simulink model "Sim2_test_cor_PI"  (R2018b)
settings: Solver=ode1  StartTime=0.0  StopTime=2  FixedStep=Time_Step  MaxStep=1e-4  RelTol=1e-3
undefined symbols (not defined in the file): abc2dq0_norm, Control_Lib, dq02abc_norm, Lg, PLL, Rg, Theta0, Time_Step, Ug, Un, V0, VSC01_id0
libraries: powerlib x35, simulink x17
(part 3 of 3)

== system Sim2_test_cor_PI/VSC02/Control loops/abc2dq0_norm1 ==
  abc : Inport
  CosSinTheta : Inport  Port=2
  Add : Sum
  Add1 : Sum  Inputs=-+
  Compare To Constant : simulink/Logic and Bit Operations/Compare To Constant  relop===  const=1  OutDataTypeStr=boolean
  Constant : Constant  Value=referenceAxisMode  OutDataTypeStr=uint16
  Demux : Demux  Outputs=2
  Demux1 : Demux  Outputs=3
  Gain : Gain  Gain=Concordia33  Multiplication=Matrix(K*u)
  Gain1 : Gain  Gain=baseUpdateGain
  Mux : Mux  Inputs=2
  Product{,1..3} (4 alike) : Product
  RotationInv90Deg : Subsystem  VariantControl=ROTATIONINV90DEG
  Switch : Switch  Criteria=u2 ~= 0
  AlphaBeta : Outport  VectorParamsAs1DForOutWhenUnconnected=off
  dq : Outport  Port=2  VectorParamsAs1DForOutWhenUnconnected=off
  ZeroSequence : Outport  Port=3  VectorParamsAs1DForOutWhenUnconnected=off
  wires:
  Gain1/1 -> Gain/1
  Compare To Constant/1 -> Switch/2
  Constant/1 -> Compare To Constant/1
  RotationInv90Deg/1(CosSinThetaOut) -> Switch/3
  CosSinTheta/1 -> RotationInv90Deg/1(CosSinThetaIn), Switch/1
  Switch/1 -> Demux/1
  Demux/1 -> Product/2, Product3/2
  Product3/1 -> Add1/2
  Product1/1 -> Add/2
  Demux/2 -> Product1/2, Product2/2
  Add1/1 -> Mux/2
  Gain/1 -> Demux1/1, AlphaBeta/1
  Demux1/2 -> Product3/1, Product1/1  "beta"
  Mux/1 -> dq/1
  Demux1/3 -> ZeroSequence/1  "zero"
  Add/1 -> Mux/1
  Demux1/1 -> Product2/1, Product/1  "alpha"
  Product/1 -> Add/1
  Product2/1 -> Add1/1
  abc/1 -> Gain1/1

== system Sim2_test_cor_PI/VSC02/Control loops/dq02abc_norm ==
  dq : Inport
  ZeroSequence : Inport  Port=2
  CosSinTheta : Inport  Port=3
  Add : Sum  Inputs=+-
  Add1 : Sum
  Compare To Constant : simulink/Logic and Bit Operations/Compare To Constant  relop===  const=1  OutDataTypeStr=boolean
  Constant : Constant  Value=referenceAxisMode  OutDataTypeStr=uint16
  Demux : Demux  Outputs=2
  Demux2 : Demux  Outputs=2
  Gain : Gain  Gain=Concordia33_inv  Multiplication=Matrix(K*u)
  Gain1 : Gain  Gain=baseUpdateGain
  Mux : Mux  Inputs=3
  Mux1 : Mux  Inputs=2
  Product{,1..3} (4 alike) : Product
  RotationInv90Deg : Subsystem  VariantControl=ROTATIONINV90DEG
  Switch : Switch  Criteria=u2 ~= 0
  AlphaBeta : Outport  VectorParamsAs1DForOutWhenUnconnected=off
  abc : Outport  Port=2  VectorParamsAs1DForOutWhenUnconnected=off
  wires:
  Gain1/1 -> abc/1
  Constant/1 -> Compare To Constant/1
  RotationInv90Deg/1(CosSinThetaOut) -> Switch/3
  Demux/1 -> Product3/2, Product/2
  Mux/1 -> Gain/1
  Switch/1 -> Demux/1
  Demux/2 -> Product2/2, Product1/2
  Mux1/1 -> AlphaBeta/1
  Product/1 -> Add/1
  Demux2/2 -> Product1/1, Product3/1  "q"
  Add1/1 -> Mux/2, Mux1/2  "beta"
  Product1/1 -> Add/2
  Compare To Constant/1 -> Switch/2
  Product2/1 -> Add1/1
  Product3/1 -> Add1/2
  CosSinTheta/1 -> Switch/1, RotationInv90Deg/1(CosSinThetaIn)
  dq/1 -> Demux2/1
  ZeroSequence/1 -> Mux/3
  Demux2/1 -> Product/1, Product2/1  "d"
  Add/1 -> Mux/1, Mux1/1  "alpha"
  Gain/1 -> Gain1/1

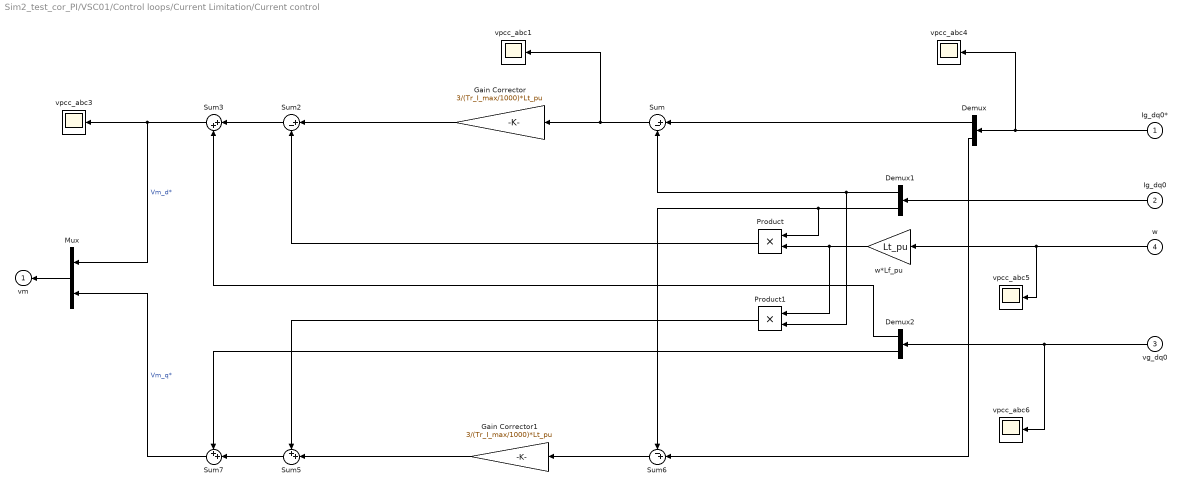
== system Sim2_test_cor_PI/VSC01/Control loops/Current Limitation/Current control ==
  Ig_dq0* : Inport
  Ig_dq0 : Inport  Port=2
  vg_dq0 : Inport  Port=3
  w : Inport  Port=4
  Demux : Demux  Outputs=2
  Demux1 : Demux  Outputs=2
  Demux2 : Demux  Outputs=2
  Gain Corrector : Gain  Gain=3/(Tr_I_max/1000)*Lt_pu
  Gain Corrector1 : Gain  Gain=3/(Tr_I_max/1000)*Lt_pu
  Mux : Mux  Inputs=2
  Product : Product  RndMeth=Zero
  Product1 : Product  RndMeth=Zero
  Sum : Sum  Inputs=|+-
  Sum2 : Sum  Inputs=|+-
  Sum3 : Sum  Inputs=|++
  Sum5 : Sum  Inputs=++|
  Sum6 : Sum  Inputs=-+|
  Sum7 : Sum  Inputs=++|
  vpcc_abc{1,3..6} (5 alike) : Scope
  w*Lf_pu : Gain  Gain=Lt_pu
  vm : Outport  InitialOutput=0  VectorParamsAs1DForOutWhenUnconnected=off
  wires:
  Demux2/2 -> Sum7/1
  Demux2/1 -> Sum3/2
  w/1 -> vpcc_abc5/1, w*Lf_pu/1
  Sum/1 -> vpcc_abc1/1, Gain Corrector/1
  Sum7/1 -> Mux/2  "Vm_q*"
  Sum3/1 -> Mux/1, vpcc_abc3/1  "Vm_d*"
  Sum5/1 -> Sum7/2
  Product1/1 -> Sum5/1
  Gain Corrector1/1 -> Sum5/2
  Demux/2 -> Sum6/2
  Sum2/1 -> Sum3/1
  Product/1 -> Sum2/2
  Demux1/2 -> Sum6/1, Product/1
  w*Lf_pu/1 -> Product/2, Product1/1
  Gain Corrector/1 -> Sum2/1
  Demux1/1 -> Sum/2, Product1/2
  Demux/1 -> Sum/1
  Ig_dq0/1 -> Demux1/1
  vg_dq0/1 -> Demux2/1, vpcc_abc6/1
  Sum6/1 -> Gain Corrector1/1
  Ig_dq0*/1 -> vpcc_abc4/1, Demux/1
  Mux/1 -> vm/1

== system Sim2_test_cor_PI/VSC01/Control loops/Current Limitation/Inverse Current control ==
  Vm_dq* : Inport
  Ig_dq : Inport  Port=2
  vg_dq : Inport  Port=3
  w : Inport  Port=4
  Demux : Demux  Outputs=2
  Demux1 : Demux  Outputs=2
  Demux2 : Demux  Outputs=2
  Gain Corrector2 : Gain  Gain=1/(3/(Tr_I_max/1000)*Lt_pu)
  Gain Corrector3 : Gain  Gain=1/(3/(Tr_I_max/1000)*Lt_pu)
  Mux : Mux  Inputs=2
  Product : Product  RndMeth=Zero
  Product1 : Product  RndMeth=Zero
  Sum : Sum  Inputs=|+-
  Sum2 : Sum  Inputs=|++
  Sum3 : Sum  Inputs=|++
  Sum5 : Sum  Inputs=-+|
  Sum6 : Sum  Inputs=-+|
  Sum7 : Sum  Inputs=++|
  w*Lf_pu : Gain  Gain=Lt_pu
  Is_dq* : Outport  InitialOutput=0  VectorParamsAs1DForOutWhenUnconnected=off
  wires:
  vg_dq/1 -> Demux2/1
  Ig_dq/1 -> Demux1/1
  Vm_dq*/1 -> Demux/1
  Demux/1 -> Sum/1
  Demux1/1 -> Sum3/2, Product1/2
  Sum/1 -> Sum2/1
  w*Lf_pu/1 -> Product1/1, Product/2
  Product/1 -> Sum2/2
  Sum2/1 -> Gain Corrector3/1
  Mux/1 -> Is_dq*/1
  Demux/2 -> Sum6/2
  Sum6/1 -> Sum5/2
  Sum5/1 -> Gain Corrector2/1
  Sum3/1 -> Mux/1  "is_d*"
  Sum7/1 -> Mux/2  "is_q*"
  w/1 -> w*Lf_pu/1
  Demux1/2 -> Sum7/1, Product/1
  Gain Corrector3/1 -> Sum3/1
  Demux2/1 -> Sum/2
  Demux2/2 -> Sum6/1
  Product1/1 -> Sum5/1
  Gain Corrector2/1 -> Sum7/2

== system Sim2_test_cor_PI/VSC01/Control loops/PLL/PI PLL controller ==
  vq : Inport
  0 - Vd1 : Gain  Gain=Kp_PLL  SaturateOnIntegerOverflow=on  OutDataTypeStr=Inherit: Same as input  ParamDataTypeStr=Inherit: Same as input
  0 - Vd2 : Gain  Gain=Ki_PLL  SaturateOnIntegerOverflow=on  OutDataTypeStr=Inherit: Same as input  ParamDataTypeStr=Inherit: Same as input
  Integrator : Integrator
  Integrator1 : Integrator  InitialCondition=Theta0*pi/180
  Sum : Sum  SaturateOnIntegerOverflow=on
  Sum1 : Sum  SaturateOnIntegerOverflow=on
  w_PLL_pu : Gain  Gain=wb  SaturateOnIntegerOverflow=on  OutDataTypeStr=Inherit: Same as input  ParamDataTypeStr=Inherit: Same as input
  w_set : Constant
  w : Outport  VectorParamsAs1DForOutWhenUnconnected=off
  Theta : Outport  Port=2  VectorParamsAs1DForOutWhenUnconnected=off
  wires:
  Integrator1/1 -> Theta/1
  0 - Vd2/1 -> Integrator/1
  w_set/1 -> Sum1/1
  w_PLL_pu/1 -> Integrator1/1
  Integrator/1 -> Sum/2
  Sum/1 -> Sum1/2
  0 - Vd1/1 -> Sum/1
  vq/1 -> 0 - Vd2/1, 0 - Vd1/1
  Sum1/1 -> w/1, w_PLL_pu/1

== system Sim2_test_cor_PI/VSC01/Control loops/PLL/abc2dq0_norm ==
  abc : Inport
  CosSinTheta : Inport  Port=2
  Add : Sum
  Add1 : Sum  Inputs=-+
  Compare To Constant : simulink/Logic and Bit Operations/Compare To Constant  relop===  const=1  OutDataTypeStr=boolean
  Constant : Constant  Value=referenceAxisMode  OutDataTypeStr=uint16
  Demux : Demux  Outputs=2
  Demux1 : Demux  Outputs=3
  Gain : Gain  Gain=Concordia33  Multiplication=Matrix(K*u)
  Gain1 : Gain  Gain=baseUpdateGain
  Mux : Mux  Inputs=2
  Product{,1..3} (4 alike) : Product
  RotationInv90Deg : Subsystem  VariantControl=ROTATIONINV90DEG
  Switch : Switch  Criteria=u2 ~= 0
  AlphaBeta : Outport  VectorParamsAs1DForOutWhenUnconnected=off
  dq : Outport  Port=2  VectorParamsAs1DForOutWhenUnconnected=off
  ZeroSequence : Outport  Port=3  VectorParamsAs1DForOutWhenUnconnected=off
  wires:
  Gain1/1 -> Gain/1
  Compare To Constant/1 -> Switch/2
  Constant/1 -> Compare To Constant/1
  RotationInv90Deg/1(CosSinThetaOut) -> Switch/3
  CosSinTheta/1 -> RotationInv90Deg/1(CosSinThetaIn), Switch/1
  Switch/1 -> Demux/1
  Demux/1 -> Product/2, Product3/2
  Product3/1 -> Add1/2
  Product1/1 -> Add/2
  Demux/2 -> Product1/2, Product2/2
  Add1/1 -> Mux/2
  Gain/1 -> Demux1/1, AlphaBeta/1
  Demux1/2 -> Product3/1, Product1/1  "beta"
  Mux/1 -> dq/1
  Demux1/3 -> ZeroSequence/1  "zero"
  Add/1 -> Mux/1
  Demux1/1 -> Product2/1, Product/1  "alpha"
  Product/1 -> Add/1
  Product2/1 -> Add1/1
  abc/1 -> Gain1/1

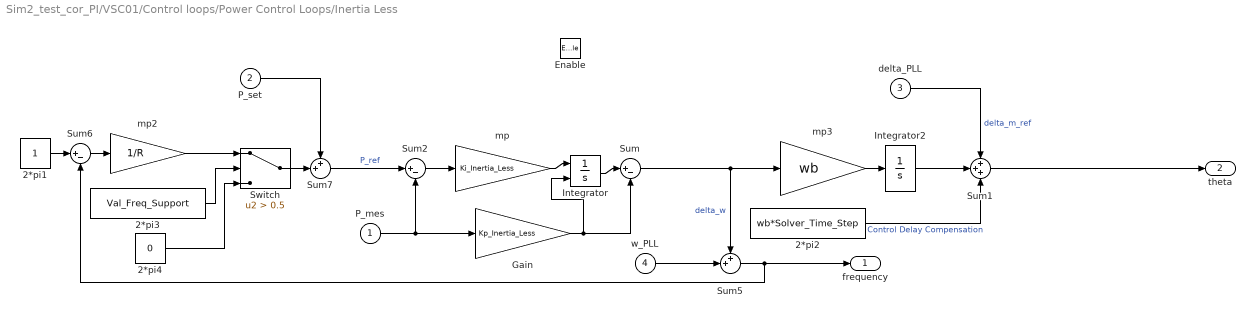
== system Sim2_test_cor_PI/VSC01/Control loops/Power Control Loops/Inertia Less ==
  P_mes : Inport
  P_set : Inport  Port=2
  delta_PLL : Inport  Port=3
  w_PLL : Inport  Port=4
  Enable : EnablePort
  2*pi1 : Constant
  2*pi2 : Constant  Value=wb*Solver_Time_Step
  2*pi3 : Constant  Value=Val_Freq_Support
  2*pi4 : Constant  Value=0
  Gain : Gain  Gain=Kp_Inertia_Less
  Integrator : Integrator  InitialConditionSource=external
  Integrator2 : Integrator  InitialCondition=(Theta_vsc0)*pi/180-Theta0*pi/180
  Sum : Sum  Inputs=|+-
  Sum1 : Sum  Inputs=+++
  Sum2 : Sum  Inputs=|+-
  Sum5 : Sum  Inputs=++|
  Sum6 : Sum  Inputs=|+-
  Sum7 : Sum  Inputs=++|
  Switch : Switch  Criteria=u2 > Threshold  Threshold=0.5
  mp : Gain  Gain=Ki_Inertia_Less
  mp2 : Gain  Gain=1/R
  mp3 : Gain  Gain=wb
  frequency : Outport  VectorParamsAs1DForOutWhenUnconnected=off
  theta : Outport  Port=2  VectorParamsAs1DForOutWhenUnconnected=off
  wires:
  Gain/1 -> Sum/2, Integrator/2
  Integrator/1 -> Sum/1
  2*pi4/1 -> Switch/3
  2*pi3/1 -> Switch/2
  mp2/1 -> Switch/1
  Integrator2/1 -> Sum1/2
  2*pi2/1 -> Sum1/3  "Control Delay Compensation"
  Sum5/1 -> Sum6/2, frequency/1
  w_PLL/1 -> Sum5/2
  delta_PLL/1 -> Sum1/1  "delta_m_ref"
  mp/1 -> Integrator/1
  mp3/1 -> Integrator2/1
  Sum/1 -> Sum5/1, mp3/1  "delta_w"
  Sum1/1 -> theta/1
  Switch/1 -> Sum7/2
  P_mes/1 -> Sum2/2, Gain/1
  Sum7/1 -> Sum2/1  "P_ref"
  P_set/1 -> Sum7/1
  Sum6/1 -> mp2/1
  2*pi1/1 -> Sum6/1
  Sum2/1 -> mp/1

== system Sim2_test_cor_PI/VSC01/Control loops/Power Control Loops/PI Controler ==
  P_mes : Inport
  P_set : Inport  Port=2
  w_set_pu : Inport  Port=3
  Enable : EnablePort
  2*pi1 : Constant
  2*pi2 : Constant  Value=wb*Solver_Time_Step
  2*pi3 : Constant  Value=Val_Freq_Support
  2*pi4 : Constant  Value=0
  Integrator : Integrator  InitialConditionSource=external
  Integrator1 : Integrator  InitialCondition=(Theta_vsc0)*pi/180
  Sum1 : Sum  Inputs=|+-
  Sum2 : Sum  Inputs=++-
  Sum3 : Sum  Inputs=|++
  Sum4 : Sum  Inputs=|++
  Sum6 : Sum  Inputs=|+-
  Switch : Switch  Criteria=u2 > Threshold  Threshold=0.5
  mp1 : Gain  Gain=wb
  mp2 : Gain  Gain=kp_GFo
  mp3 : Gain  Gain=1/(2*H_GFo)
  mp4 : Gain  Gain=1/R
  frequency : Outport  VectorParamsAs1DForOutWhenUnconnected=off
  theta : Outport  Port=2  VectorParamsAs1DForOutWhenUnconnected=off
  wires:
  Switch/1 -> Sum2/2
  2*pi4/1 -> Switch/3
  Sum6/1 -> mp4/1
  2*pi3/1 -> Switch/2
  2*pi1/1 -> Sum6/1
  mp4/1 -> Switch/1
  Sum4/1 -> Integrator/2
  mp3/1 -> Integrator/1
  mp2/1 -> Sum4/2, Sum1/2
  P_mes/1 -> mp2/1, Sum2/3
  2*pi2/1 -> Sum3/2  "Control Delay Compensation"
  mp1/1 -> Integrator1/1  "w_m"
  Sum1/1 -> Sum6/2, frequency/1, mp1/1
  Integrator/1 -> Sum1/1
  P_set/1 -> Sum2/1
  w_set_pu/1 -> Sum4/1
  Integrator1/1 -> Sum3/1  "delta_m_ref"
  Sum2/1 -> mp3/1
  Sum3/1 -> theta/1

== system Sim2_test_cor_PI/VSC01/Control loops/Power Control Loops/VSM ==
  P_mes : Inport
  P_set : Inport  Port=2
  w_PLL : Inport  Port=3
  Enable : EnablePort
  2*pi1 : Constant
  2*pi2 : Constant  Value=wb*Solver_Time_Step
  2*pi3 : Constant  Value=Val_Freq_Support
  2*pi4 : Constant  Value=0
  Gain : Gain  Gain=kd
  Gain1 : Gain  Gain=1/(2*H_GFo)
  Integrator : Integrator  InitialCondition=1
  Integrator1 : Integrator  InitialCondition=Theta_vsc0*pi/180
  Sum : Sum  Inputs=|+-
  Sum1 : Sum  Inputs=++-
  Sum3 : Sum  Inputs=|++
  Sum6 : Sum  Inputs=|+-
  Sum7 : Sum  Inputs=++|
  Switch : Switch  Criteria=u2 > Threshold  Threshold=0.5
  mp1 : Gain  Gain=1/R
  mp2 : Gain  Gain=wb
  frequency : Outport  VectorParamsAs1DForOutWhenUnconnected=off
  theta : Outport  Port=2  VectorParamsAs1DForOutWhenUnconnected=off
  wires:
  Gain1/1 -> Integrator/1
  Sum7/1 -> Sum1/2  "P_ref"
  Sum1/1 -> Gain1/1
  Gain/1 -> Sum1/1
  Sum/1 -> Gain/1
  w_PLL/1 -> Sum/1
  2*pi4/1 -> Switch/3
  2*pi3/1 -> Switch/2
  mp1/1 -> Switch/1
  2*pi1/1 -> Sum6/1
  Sum6/1 -> mp1/1
  P_set/1 -> Sum7/1
  Switch/1 -> Sum7/2
  2*pi2/1 -> Sum3/2  "Control Delay Compensation"
  mp2/1 -> Integrator1/1
  P_mes/1 -> Sum1/3
  Integrator/1 -> Sum6/2, frequency/1, mp2/1, Sum/2  "wm"
  Integrator1/1 -> Sum3/1  "delta_m_ref"
  Sum3/1 -> theta/1

== system Sim2_test_cor_PI/VSC01/Control loops/Transient Damping Resistance/Filter w_LF ==
  e : Inport
  1/T_LP : Gain  Gain=W_TVR  SaturateOnIntegerOverflow=on  OutDataTypeStr=Inherit: Same as input  ParamDataTypeStr=Inherit: Same as input
  Integrator : Integrator  InitialConditionSource=external  InitialCondition=[VSC01_id0*0.04]
  Sum1 : Sum  Inputs=|+-  InputSameDT=on  SaturateOnIntegerOverflow=on  OutDataTypeStr=Inherit: Same as first input
  s : Outport  VectorParamsAs1DForOutWhenUnconnected=off
  wires:
  e/1 -> Sum1/1, Integrator/2
  Integrator/1 -> s/1, Sum1/2
  1/T_LP/1 -> Integrator/1
  Sum1/1 -> 1/T_LP/1

== system Sim2_test_cor_PI/VSC01/Control loops/VI/dq to phasor ==
  dq_mes : Inport
  Demux : Demux  Outputs=2
      settings: DisplayOption=none
  Sqrt : Sqrt  SaturateOnIntegerOverflow=on
  Sum4 : Sum  Inputs=|++  InputSameDT=on  SaturateOnIntegerOverflow=on  OutDataTypeStr=Inherit: Same as first input
  Vrdird : Product  InputSameDT=on  RndMeth=Zero  SaturateOnIntegerOverflow=on  OutDataTypeStr=Inherit: Same as first input
  Vrqirq : Product  InputSameDT=on  RndMeth=Zero  SaturateOnIntegerOverflow=on  OutDataTypeStr=Inherit: Same as first input
  rms : Outport  VectorParamsAs1DForOutWhenUnconnected=off
  wires:
  Sum4/1 -> Sqrt/1
  Vrqirq/1 -> Sum4/2
  Vrdird/1 -> Sum4/1
  Demux/2 -> Vrqirq/2, Vrqirq/1
  Demux/1 -> Vrdird/2, Vrdird/1
  dq_mes/1 -> Demux/1
  Sqrt/1 -> rms/1

== system Sim2_test_cor_PI/VSC01/Control loops/abc2dq0_norm/RotationInv90Deg ==
  CosSinThetaIn : Inport
  Demux : Demux  Outputs=2
  Gain1 : Gain  Gain=-1
  Mux : Mux  Inputs=2
  CosSinThetaOut : Outport  VectorParamsAs1DForOutWhenUnconnected=off
  wires:
  Gain1/1 -> Mux/2
  Demux/2 -> Mux/1
  Demux/1 -> Gain1/1
  CosSinThetaIn/1 -> Demux/1
  Mux/1 -> CosSinThetaOut/1

== system Sim2_test_cor_PI/VSC01/Control loops/abc2dq0_norm1/RotationInv90Deg ==
  CosSinThetaIn : Inport
  Demux : Demux  Outputs=2
  Gain1 : Gain  Gain=-1
  Mux : Mux  Inputs=2
  CosSinThetaOut : Outport  VectorParamsAs1DForOutWhenUnconnected=off
  wires:
  Gain1/1 -> Mux/2
  Demux/2 -> Mux/1
  Demux/1 -> Gain1/1
  CosSinThetaIn/1 -> Demux/1
  Mux/1 -> CosSinThetaOut/1

== system Sim2_test_cor_PI/VSC01/Control loops/dq02abc_norm/RotationInv90Deg ==
  CosSinThetaIn : Inport
  Demux1 : Demux  Outputs=2
  Gain1 : Gain  Gain=-1
  Mux1 : Mux  Inputs=2
  CosSinThetaOut : Outport  VectorParamsAs1DForOutWhenUnconnected=off
  wires:
  Demux1/2 -> Mux1/1
  CosSinThetaIn/1 -> Demux1/1
  Mux1/1 -> CosSinThetaOut/1
  Demux1/1 -> Gain1/1
  Gain1/1 -> Mux1/2

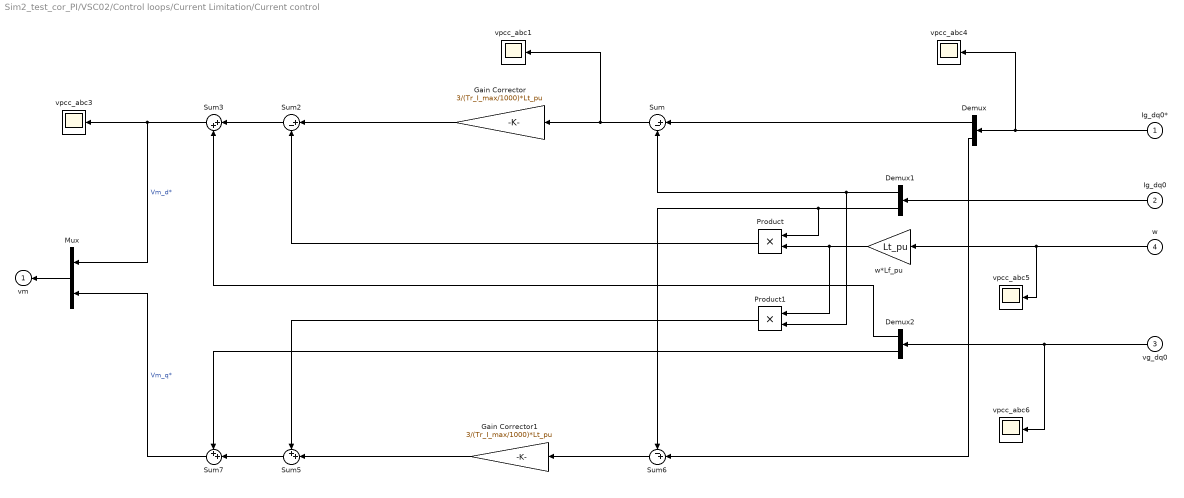
== system Sim2_test_cor_PI/VSC02/Control loops/Current Limitation/Current control ==
  Ig_dq0* : Inport
  Ig_dq0 : Inport  Port=2
  vg_dq0 : Inport  Port=3
  w : Inport  Port=4
  Demux : Demux  Outputs=2
  Demux1 : Demux  Outputs=2
  Demux2 : Demux  Outputs=2
  Gain Corrector : Gain  Gain=3/(Tr_I_max/1000)*Lt_pu
  Gain Corrector1 : Gain  Gain=3/(Tr_I_max/1000)*Lt_pu
  Mux : Mux  Inputs=2
  Product : Product  RndMeth=Zero
  Product1 : Product  RndMeth=Zero
  Sum : Sum  Inputs=|+-
  Sum2 : Sum  Inputs=|+-
  Sum3 : Sum  Inputs=|++
  Sum5 : Sum  Inputs=++|
  Sum6 : Sum  Inputs=-+|
  Sum7 : Sum  Inputs=++|
  vpcc_abc{1,3..6} (5 alike) : Scope
  w*Lf_pu : Gain  Gain=Lt_pu
  vm : Outport  InitialOutput=0  VectorParamsAs1DForOutWhenUnconnected=off
  wires:
  Demux2/2 -> Sum7/1
  Demux2/1 -> Sum3/2
  w/1 -> vpcc_abc5/1, w*Lf_pu/1
  Sum/1 -> vpcc_abc1/1, Gain Corrector/1
  Sum7/1 -> Mux/2  "Vm_q*"
  Sum3/1 -> Mux/1, vpcc_abc3/1  "Vm_d*"
  Sum5/1 -> Sum7/2
  Product1/1 -> Sum5/1
  Gain Corrector1/1 -> Sum5/2
  Demux/2 -> Sum6/2
  Sum2/1 -> Sum3/1
  Product/1 -> Sum2/2
  Demux1/2 -> Sum6/1, Product/1
  w*Lf_pu/1 -> Product/2, Product1/1
  Gain Corrector/1 -> Sum2/1
  Demux1/1 -> Sum/2, Product1/2
  Demux/1 -> Sum/1
  Ig_dq0/1 -> Demux1/1
  vg_dq0/1 -> Demux2/1, vpcc_abc6/1
  Sum6/1 -> Gain Corrector1/1
  Ig_dq0*/1 -> vpcc_abc4/1, Demux/1
  Mux/1 -> vm/1

== system Sim2_test_cor_PI/VSC02/Control loops/Current Limitation/Inverse Current control ==
  Vm_dq* : Inport
  Ig_dq : Inport  Port=2
  vg_dq : Inport  Port=3
  w : Inport  Port=4
  Demux : Demux  Outputs=2
  Demux1 : Demux  Outputs=2
  Demux2 : Demux  Outputs=2
  Gain Corrector2 : Gain  Gain=1/(3/(Tr_I_max/1000)*Lt_pu)
  Gain Corrector3 : Gain  Gain=1/(3/(Tr_I_max/1000)*Lt_pu)
  Mux : Mux  Inputs=2
  Product : Product  RndMeth=Zero
  Product1 : Product  RndMeth=Zero
  Sum : Sum  Inputs=|+-
  Sum2 : Sum  Inputs=|++
  Sum3 : Sum  Inputs=|++
  Sum5 : Sum  Inputs=-+|
  Sum6 : Sum  Inputs=-+|
  Sum7 : Sum  Inputs=++|
  w*Lf_pu : Gain  Gain=Lt_pu
  Is_dq* : Outport  InitialOutput=0  VectorParamsAs1DForOutWhenUnconnected=off
  wires:
  vg_dq/1 -> Demux2/1
  Ig_dq/1 -> Demux1/1
  Vm_dq*/1 -> Demux/1
  Demux/1 -> Sum/1
  Demux1/1 -> Sum3/2, Product1/2
  Sum/1 -> Sum2/1
  w*Lf_pu/1 -> Product1/1, Product/2
  Product/1 -> Sum2/2
  Sum2/1 -> Gain Corrector3/1
  Mux/1 -> Is_dq*/1
  Demux/2 -> Sum6/2
  Sum6/1 -> Sum5/2
  Sum5/1 -> Gain Corrector2/1
  Sum3/1 -> Mux/1  "is_d*"
  Sum7/1 -> Mux/2  "is_q*"
  w/1 -> w*Lf_pu/1
  Demux1/2 -> Sum7/1, Product/1
  Gain Corrector3/1 -> Sum3/1
  Demux2/1 -> Sum/2
  Demux2/2 -> Sum6/1
  Product1/1 -> Sum5/1
  Gain Corrector2/1 -> Sum7/2

== system Sim2_test_cor_PI/VSC02/Control loops/PLL/PI PLL controller ==
  vq : Inport
  0 - Vd1 : Gain  Gain=Kp_PLL  SaturateOnIntegerOverflow=on  OutDataTypeStr=Inherit: Same as input  ParamDataTypeStr=Inherit: Same as input
  0 - Vd2 : Gain  Gain=Ki_PLL  SaturateOnIntegerOverflow=on  OutDataTypeStr=Inherit: Same as input  ParamDataTypeStr=Inherit: Same as input
  Integrator : Integrator
  Integrator1 : Integrator  InitialCondition=Theta0*pi/180
  Sum : Sum  SaturateOnIntegerOverflow=on
  Sum1 : Sum  SaturateOnIntegerOverflow=on
  w_PLL_pu : Gain  Gain=wb  SaturateOnIntegerOverflow=on  OutDataTypeStr=Inherit: Same as input  ParamDataTypeStr=Inherit: Same as input
  w_set : Constant
  w : Outport  VectorParamsAs1DForOutWhenUnconnected=off
  Theta : Outport  Port=2  VectorParamsAs1DForOutWhenUnconnected=off
  wires:
  Integrator1/1 -> Theta/1
  0 - Vd2/1 -> Integrator/1
  w_set/1 -> Sum1/1
  w_PLL_pu/1 -> Integrator1/1
  Integrator/1 -> Sum/2
  Sum/1 -> Sum1/2
  0 - Vd1/1 -> Sum/1
  vq/1 -> 0 - Vd2/1, 0 - Vd1/1
  Sum1/1 -> w/1, w_PLL_pu/1

== system Sim2_test_cor_PI/VSC02/Control loops/PLL/abc2dq0_norm ==
  abc : Inport
  CosSinTheta : Inport  Port=2
  Add : Sum
  Add1 : Sum  Inputs=-+
  Compare To Constant : simulink/Logic and Bit Operations/Compare To Constant  relop===  const=1  OutDataTypeStr=boolean
  Constant : Constant  Value=referenceAxisMode  OutDataTypeStr=uint16
  Demux : Demux  Outputs=2
  Demux1 : Demux  Outputs=3
  Gain : Gain  Gain=Concordia33  Multiplication=Matrix(K*u)
  Gain1 : Gain  Gain=baseUpdateGain
  Mux : Mux  Inputs=2
  Product{,1..3} (4 alike) : Product
  RotationInv90Deg : Subsystem  VariantControl=ROTATIONINV90DEG
  Switch : Switch  Criteria=u2 ~= 0
  AlphaBeta : Outport  VectorParamsAs1DForOutWhenUnconnected=off
  dq : Outport  Port=2  VectorParamsAs1DForOutWhenUnconnected=off
  ZeroSequence : Outport  Port=3  VectorParamsAs1DForOutWhenUnconnected=off
  wires:
  Gain1/1 -> Gain/1
  Compare To Constant/1 -> Switch/2
  Constant/1 -> Compare To Constant/1
  RotationInv90Deg/1(CosSinThetaOut) -> Switch/3
  CosSinTheta/1 -> RotationInv90Deg/1(CosSinThetaIn), Switch/1
  Switch/1 -> Demux/1
  Demux/1 -> Product/2, Product3/2
  Product3/1 -> Add1/2
  Product1/1 -> Add/2
  Demux/2 -> Product1/2, Product2/2
  Add1/1 -> Mux/2
  Gain/1 -> Demux1/1, AlphaBeta/1
  Demux1/2 -> Product3/1, Product1/1  "beta"
  Mux/1 -> dq/1
  Demux1/3 -> ZeroSequence/1  "zero"
  Add/1 -> Mux/1
  Demux1/1 -> Product2/1, Product/1  "alpha"
  Product/1 -> Add/1
  Product2/1 -> Add1/1
  abc/1 -> Gain1/1

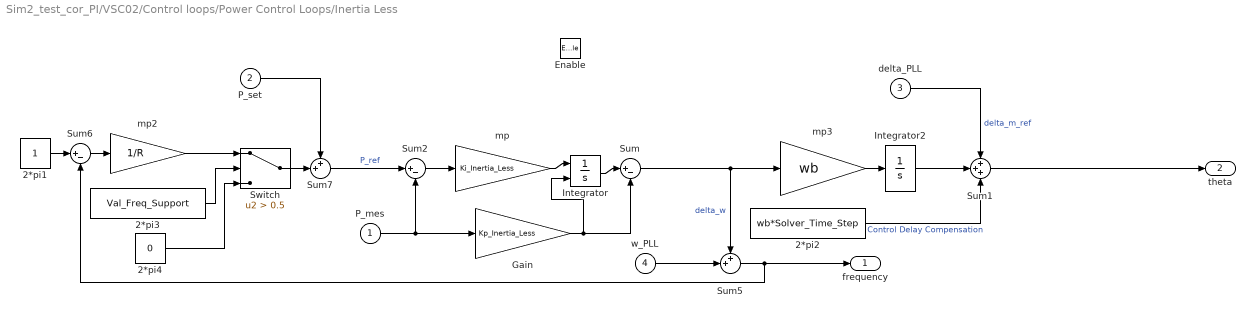
== system Sim2_test_cor_PI/VSC02/Control loops/Power Control Loops/Inertia Less ==
  P_mes : Inport
  P_set : Inport  Port=2
  delta_PLL : Inport  Port=3
  w_PLL : Inport  Port=4
  Enable : EnablePort
  2*pi1 : Constant
  2*pi2 : Constant  Value=wb*Solver_Time_Step
  2*pi3 : Constant  Value=Val_Freq_Support
  2*pi4 : Constant  Value=0
  Gain : Gain  Gain=Kp_Inertia_Less
  Integrator : Integrator  InitialConditionSource=external
  Integrator2 : Integrator  InitialCondition=(Theta_vsc0)*pi/180-Theta0*pi/180
  Sum : Sum  Inputs=|+-
  Sum1 : Sum  Inputs=+++
  Sum2 : Sum  Inputs=|+-
  Sum5 : Sum  Inputs=++|
  Sum6 : Sum  Inputs=|+-
  Sum7 : Sum  Inputs=++|
  Switch : Switch  Criteria=u2 > Threshold  Threshold=0.5
  mp : Gain  Gain=Ki_Inertia_Less
  mp2 : Gain  Gain=1/R
  mp3 : Gain  Gain=wb
  frequency : Outport  VectorParamsAs1DForOutWhenUnconnected=off
  theta : Outport  Port=2  VectorParamsAs1DForOutWhenUnconnected=off
  wires:
  Gain/1 -> Sum/2, Integrator/2
  Integrator/1 -> Sum/1
  2*pi4/1 -> Switch/3
  2*pi3/1 -> Switch/2
  mp2/1 -> Switch/1
  Integrator2/1 -> Sum1/2
  2*pi2/1 -> Sum1/3  "Control Delay Compensation"
  Sum5/1 -> Sum6/2, frequency/1
  w_PLL/1 -> Sum5/2
  delta_PLL/1 -> Sum1/1  "delta_m_ref"
  mp/1 -> Integrator/1
  mp3/1 -> Integrator2/1
  Sum/1 -> Sum5/1, mp3/1  "delta_w"
  Sum1/1 -> theta/1
  Switch/1 -> Sum7/2
  P_mes/1 -> Sum2/2, Gain/1
  Sum7/1 -> Sum2/1  "P_ref"
  P_set/1 -> Sum7/1
  Sum6/1 -> mp2/1
  2*pi1/1 -> Sum6/1
  Sum2/1 -> mp/1

== system Sim2_test_cor_PI/VSC02/Control loops/Power Control Loops/PI Controler ==
  P_mes : Inport
  P_set : Inport  Port=2
  w_set_pu : Inport  Port=3
  Enable : EnablePort
  2*pi1 : Constant
  2*pi2 : Constant  Value=wb*Solver_Time_Step
  2*pi3 : Constant  Value=Val_Freq_Support
  2*pi4 : Constant  Value=0
  Integrator : Integrator  InitialConditionSource=external
  Integrator1 : Integrator  InitialCondition=(Theta_vsc0)*pi/180
  Sum1 : Sum  Inputs=|+-
  Sum2 : Sum  Inputs=++-
  Sum3 : Sum  Inputs=|++
  Sum4 : Sum  Inputs=|++
  Sum6 : Sum  Inputs=|+-
  Switch : Switch  Criteria=u2 > Threshold  Threshold=0.5
  mp1 : Gain  Gain=wb
  mp2 : Gain  Gain=kp_GFo
  mp3 : Gain  Gain=1/(2*H_GFo)
  mp4 : Gain  Gain=1/R
  frequency : Outport  VectorParamsAs1DForOutWhenUnconnected=off
  theta : Outport  Port=2  VectorParamsAs1DForOutWhenUnconnected=off
  wires:
  Switch/1 -> Sum2/2
  2*pi4/1 -> Switch/3
  Sum6/1 -> mp4/1
  2*pi3/1 -> Switch/2
  2*pi1/1 -> Sum6/1
  mp4/1 -> Switch/1
  Sum4/1 -> Integrator/2
  mp3/1 -> Integrator/1
  mp2/1 -> Sum4/2, Sum1/2
  P_mes/1 -> mp2/1, Sum2/3
  2*pi2/1 -> Sum3/2  "Control Delay Compensation"
  mp1/1 -> Integrator1/1  "w_m"
  Sum1/1 -> Sum6/2, frequency/1, mp1/1
  Integrator/1 -> Sum1/1
  P_set/1 -> Sum2/1
  w_set_pu/1 -> Sum4/1
  Integrator1/1 -> Sum3/1  "delta_m_ref"
  Sum2/1 -> mp3/1
  Sum3/1 -> theta/1

== system Sim2_test_cor_PI/VSC02/Control loops/Power Control Loops/VSM ==
  P_mes : Inport
  P_set : Inport  Port=2
  w_PLL : Inport  Port=3
  Enable : EnablePort
  2*pi1 : Constant
  2*pi2 : Constant  Value=wb*Solver_Time_Step
  2*pi3 : Constant  Value=Val_Freq_Support
  2*pi4 : Constant  Value=0
  Gain : Gain  Gain=kd
  Gain1 : Gain  Gain=1/(2*H_GFo)
  Integrator : Integrator  InitialCondition=1
  Integrator1 : Integrator  InitialCondition=Theta_vsc0*pi/180
  Sum : Sum  Inputs=|+-
  Sum1 : Sum  Inputs=++-
  Sum3 : Sum  Inputs=|++
  Sum6 : Sum  Inputs=|+-
  Sum7 : Sum  Inputs=++|
  Switch : Switch  Criteria=u2 > Threshold  Threshold=0.5
  mp1 : Gain  Gain=1/R
  mp2 : Gain  Gain=wb
  frequency : Outport  VectorParamsAs1DForOutWhenUnconnected=off
  theta : Outport  Port=2  VectorParamsAs1DForOutWhenUnconnected=off
  wires:
  Gain1/1 -> Integrator/1
  Sum7/1 -> Sum1/2  "P_ref"
  Sum1/1 -> Gain1/1
  Gain/1 -> Sum1/1
  Sum/1 -> Gain/1
  w_PLL/1 -> Sum/1
  2*pi4/1 -> Switch/3
  2*pi3/1 -> Switch/2
  mp1/1 -> Switch/1
  2*pi1/1 -> Sum6/1
  Sum6/1 -> mp1/1
  P_set/1 -> Sum7/1
  Switch/1 -> Sum7/2
  2*pi2/1 -> Sum3/2  "Control Delay Compensation"
  mp2/1 -> Integrator1/1
  P_mes/1 -> Sum1/3
  Integrator/1 -> Sum6/2, frequency/1, mp2/1, Sum/2  "wm"
  Integrator1/1 -> Sum3/1  "delta_m_ref"
  Sum3/1 -> theta/1

== system Sim2_test_cor_PI/VSC02/Control loops/Transient Damping Resistance/Filter w_LF ==
  e : Inport
  1/T_LP : Gain  Gain=W_TVR  SaturateOnIntegerOverflow=on  OutDataTypeStr=Inherit: Same as input  ParamDataTypeStr=Inherit: Same as input
  Integrator : Integrator  InitialConditionSource=external  InitialCondition=[VSC01_id0*0.04]
  Sum1 : Sum  Inputs=|+-  InputSameDT=on  SaturateOnIntegerOverflow=on  OutDataTypeStr=Inherit: Same as first input
  s : Outport  VectorParamsAs1DForOutWhenUnconnected=off
  wires:
  e/1 -> Sum1/1, Integrator/2
  Integrator/1 -> s/1, Sum1/2
  1/T_LP/1 -> Integrator/1
  Sum1/1 -> 1/T_LP/1

== system Sim2_test_cor_PI/VSC02/Control loops/VI/dq to phasor ==
  dq_mes : Inport
  Demux : Demux  Outputs=2
      settings: DisplayOption=none
  Sqrt : Sqrt  SaturateOnIntegerOverflow=on
  Sum4 : Sum  Inputs=|++  InputSameDT=on  SaturateOnIntegerOverflow=on  OutDataTypeStr=Inherit: Same as first input
  Vrdird : Product  InputSameDT=on  RndMeth=Zero  SaturateOnIntegerOverflow=on  OutDataTypeStr=Inherit: Same as first input
  Vrqirq : Product  InputSameDT=on  RndMeth=Zero  SaturateOnIntegerOverflow=on  OutDataTypeStr=Inherit: Same as first input
  rms : Outport  VectorParamsAs1DForOutWhenUnconnected=off
  wires:
  Sum4/1 -> Sqrt/1
  Vrqirq/1 -> Sum4/2
  Vrdird/1 -> Sum4/1
  Demux/2 -> Vrqirq/2, Vrqirq/1
  Demux/1 -> Vrdird/2, Vrdird/1
  dq_mes/1 -> Demux/1
  Sqrt/1 -> rms/1

== system Sim2_test_cor_PI/VSC02/Control loops/abc2dq0_norm/RotationInv90Deg ==
  CosSinThetaIn : Inport
  Demux : Demux  Outputs=2
  Gain1 : Gain  Gain=-1
  Mux : Mux  Inputs=2
  CosSinThetaOut : Outport  VectorParamsAs1DForOutWhenUnconnected=off
  wires:
  Gain1/1 -> Mux/2
  Demux/2 -> Mux/1
  Demux/1 -> Gain1/1
  CosSinThetaIn/1 -> Demux/1
  Mux/1 -> CosSinThetaOut/1

== system Sim2_test_cor_PI/VSC02/Control loops/abc2dq0_norm1/RotationInv90Deg ==
  CosSinThetaIn : Inport
  Demux : Demux  Outputs=2
  Gain1 : Gain  Gain=-1
  Mux : Mux  Inputs=2
  CosSinThetaOut : Outport  VectorParamsAs1DForOutWhenUnconnected=off
  wires:
  Gain1/1 -> Mux/2
  Demux/2 -> Mux/1
  Demux/1 -> Gain1/1
  CosSinThetaIn/1 -> Demux/1
  Mux/1 -> CosSinThetaOut/1

== system Sim2_test_cor_PI/VSC02/Control loops/dq02abc_norm/RotationInv90Deg ==
  CosSinThetaIn : Inport
  Demux1 : Demux  Outputs=2
  Gain1 : Gain  Gain=-1
  Mux1 : Mux  Inputs=2
  CosSinThetaOut : Outport  VectorParamsAs1DForOutWhenUnconnected=off
  wires:
  Demux1/2 -> Mux1/1
  CosSinThetaIn/1 -> Demux1/1
  Mux1/1 -> CosSinThetaOut/1
  Demux1/1 -> Gain1/1
  Gain1/1 -> Mux1/2

== system Sim2_test_cor_PI/VSC01/Control loops/PLL/abc2dq0_norm/RotationInv90Deg ==
  CosSinThetaIn : Inport
  Demux : Demux  Outputs=2
  Gain1 : Gain  Gain=-1
  Mux : Mux  Inputs=2
  CosSinThetaOut : Outport  VectorParamsAs1DForOutWhenUnconnected=off
  wires:
  Gain1/1 -> Mux/2
  Demux/2 -> Mux/1
  Demux/1 -> Gain1/1
  CosSinThetaIn/1 -> Demux/1
  Mux/1 -> CosSinThetaOut/1

== system Sim2_test_cor_PI/VSC02/Control loops/PLL/abc2dq0_norm/RotationInv90Deg ==
  CosSinThetaIn : Inport
  Demux : Demux  Outputs=2
  Gain1 : Gain  Gain=-1
  Mux : Mux  Inputs=2
  CosSinThetaOut : Outport  VectorParamsAs1DForOutWhenUnconnected=off
  wires:
  Gain1/1 -> Mux/2
  Demux/2 -> Mux/1
  Demux/1 -> Gain1/1
  CosSinThetaIn/1 -> Demux/1
  Mux/1 -> CosSinThetaOut/1
